simulink library "Tire_Models"  (R2020b)
settings: Solver=VariableStepAuto  StartTime=0.0  StopTime=10.0  RelTol=1e-3
undefined symbols (not defined in the file): Vehicle, X, Y, Z
libraries: Tire_Delft x4, Tire_CFL x2, Tire_MFEval x2, Tire_MFSwift x2, Tire_Testrig_Post x2, $bdroot x2, sm_lib x2
Description:
  | Copyright 2020 The MathWorks, Inc.
settings Model: Creator=smiller  LastModifiedBy=smiller
settings DataIOCC: ReturnWorkspaceOutputs=off
settings DebuggingCC: ArithmeticOperatorsInVariantConditions=warning
settings SFSimCC: CustomCodeUndefinedFunction=UseInterfaceOnly

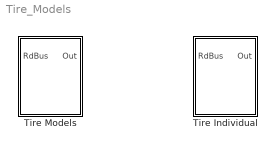
== system Tire_Models ==
  Tire Individual : Subsystem  Tag=PublishSubsystem  Variant=on  VariantControlMode=label  VariantControl=Variant1  LabelModeActiveChoice=MFEval  mask(Tire){popup_leftRight=Right, tir_index=1, Tire=Vehicle.Chassis.TireF, VariantLabel=Vehicle.Chassis.TireF.class.Value, InitTriggerDropdown=1}
      mask prompts: popup_leftRight "Left/Right"; tir_index "Tire Index"; Tire "Tire Parameters"; VariantLabel "Variant Label"; InitTriggerDropdown "Initialization Trigger Dropdown"
      mask help: Configurable tire model.
      mask init:
      | curblk = gcb;
      | 
      | % Set variant for this block
      | set_param(curblk,'LabelModeActiveChoice',VariantLabel);
      | 
      | tir_variant = get_param(gcb,'ActiveVariant');
      | if (popup_leftRight == 1)
      |     if(strcmp(tir_variant,'MFEval'))
      |         set_param([gcb '/MFEval'],'tir_side','1 left');
      |         set_param([gcb '/MFEval'],'popup_leftRight','Left');
      |     elseif(strcmp(tir_variant,'CFL'))
      |         set_param([gcb '/CFL'],'popup_leftRight','Left');
      |     elseif(strcmp(tir_variant,'Testrig_Post'))
      |         set_param([gcb '/Testrig Post'],'popup_leftRight','Left');
      |     elseif(strcmp(tir_variant,'Delft'))
      |         set_param([gcb '/Delft'],'tire_side_mode','(1xxx) left');
      |         set_param([gcb '/Delft'],'popup_leftRight','Left');
      |     elseif(strcmp(tir_variant,'MFSwift'))
      |         set_param([gcb '/MFSwift'],'tire_side_mode','(x1xxx) left');
      |         set_param([gcb '/MFSwift'],'popup_leftRight','Left');    
      |     end
      | elseif (popup_leftRight == 2)
      |     if(strcmp(tir_variant,'MFEval'))
      |         set_param([gcb '/MFEval'],'tir_side','2 right');
      |         set_param([gcb '/MFEval'],'popup_leftRight','Right');
      |     elseif(strcmp(tir_variant,'CFL'))
      |         set_param([gcb '/CFL'],'popup_leftRight','Right');
      |     elseif(strcmp(tir_variant,'Testrig_Post'))
      |         set_param([gcb '/Testrig Post'],'popup_leftRight','Right');        
      |     elseif(strcmp(tir_variant,'Delft'))
      |         set_param([gcb '/Delft'],'tire_side_mode','(2xxx) right');
      |         set_param([gcb '/Delft'],'popup_leftRight','Right');
      |     elseif(strcmp(tir_variant,'MFSwift'))
      |         set_param([gcb '/MFSwift'],'tire_side_mode','(x2xxx) right');
      |         set_param([gcb '/MFSwift'],'popup_leftRight','Right');    
      |     end
      | end
      | 
      | % Trigger Mask Initialization for
      | % variant subsystems below this level
      | sm_car_lib_maskInitTrigger(curblk);
      settings: AttributesFormatString=%<ActiveVariant>
      mask TypeOptions popup_leftRight: Left | Right
      mask TypeOptions InitTriggerDropdown: 0 | 1
      mask Display:
      | switch lower(get_param(gcb,'LabelModeActiveChoice'))
      |     case 'mfeval', image('sm_car_vehicle_tire_mfeval_IMAGE.png');
      |     case 'delft', image('sm_car_vehicle_tire_delft_IMAGE.png');
      |     case 'mfswift', image('sm_car_vehicle_tire_delft_IMAGE.png');
      |     case 'cpi', image('sm_car_vehicle_tire_delftcpi_IMAGE.png');
      |     case 'cfl', image('sm_car_vehicle_tire_cfl_IMAGE.png');
      |     case 'testrig_post', image('sm_car_vehicle_tire_testrig_IMAGE.png');
      | end
  Tire Models : Subsystem  Tag=PublishSubsystem  Variant=on  VariantControlMode=label  VariantControl=Variant1  LabelModeActiveChoice=MFEval  mask(Tire){popup_leftRight=Right, tir_index=1, Tire=Vehicle.Chassis.TireR, VariantLabel=Vehicle.Chassis.TireR.class.Value, InitTriggerDropdown=1}
      mask prompts: popup_leftRight "Left/Right"; tir_index "Tire Index"; Tire "Tire Parameters"; VariantLabel "Variant Label"; InitTriggerDropdown "Initialization Trigger Dropdown"
      mask help: Configurable tire model.
      mask init:
      | curblk = gcb;
      | 
      | % Set variant for this block 
      | set_param(curblk,'LabelModeActiveChoice',VariantLabel);
      | 
      | tir_variant = get_param(gcb,'ActiveVariant');
      | if (popup_leftRight == 1)
      |     rhs_tire = 1;
      |     if(strcmp(tir_variant,'MFEval'))
      |         set_param([gcb '/MFEval'],'tir_side','1 left');
      |         set_param([gcb '/MFEval'],'popup_leftRight','Left');
      |     elseif(strcmp(tir_variant,'Tire2x'))
      |         set_param([gcb '/Tire2x'],'popup_leftRight','Left');
      |     elseif(strcmp(tir_variant,'CFL'))
      |         set_param([gcb '/CFL'],'popup_leftRight','Left');
      |     elseif(strcmp(tir_variant,'Testrig_Post'))
      |         set_param([gcb '/Testrig Post'],'popup_leftRight','Left');
      |     elseif(strcmp(tir_variant,'Delft'))
      |         set_param([gcb '/Delft'],'tire_side_mode','(1xxx) left');
      |         set_param([gcb '/Delft'],'popup_leftRight','Left');
      |     elseif(strcmp(tir_variant,'MFSwift'))
      |         set_param([gcb '/MFSwift'],'tire_side_mode','(x1xxx) left');
      |         set_param([gcb '/MFSwift'],'popup_leftRight','Left');
      |     end
      | elseif (popup_leftRight == 2)
      |     rhs_tire = -1;
      |     if(strcmp(tir_variant,'MFEval'))
      |         set_param([gcb '/MFEval'],'tir_side','2 right');
      |         set_param([gcb '/MFEval'],'popup_leftRight','Right');
      |     elseif(strcmp(tir_variant,'Tire2x'))
      |         set_param([gcb '/Tire2x'],'popup_leftRight','Right');
      |     elseif(strcmp(tir_variant,'CFL'))
      |         set_param([gcb '/CFL'],'popup_leftRight','Right');
      |     elseif(strcmp(tir_variant,'Testrig_Post'))
      |         set_param([gcb '/Testrig Post'],'popup_leftRight','Right');
      |     elseif(strcmp(tir_variant,'Delft'))
      |         set_param([gcb '/Delft'],'tire_side_mode','(2xxx) right');
      |         set_param([gcb '/Delft'],'popup_leftRight','Right');
      |     elseif(strcmp(tir_variant,'MFSwift'))
      |         set_param([gcb '/MFSwift'],'tire_side_mode','(x2xxx) right');
      |         set_param([gcb '/MFSwift'],'popup_leftRight','Right');
      |     end
      | end
      | 
      | % Trigger Mask Initialization for 
      | % variant subsystems below this level
      | sm_car_lib_maskInitTrigger(curblk);
      settings: AttributesFormatString=%<ActiveVariant>
      mask TypeOptions popup_leftRight: Left | Right
      mask TypeOptions InitTriggerDropdown: 0 | 1
      mask Display:
      | switch lower(get_param(gcb,'LabelModeActiveChoice'))
      |     case 'mfeval', image('sm_car_vehicle_tire_mfeval_IMAGE.png');
      |     case 'delft', image('sm_car_vehicle_tire_delft_IMAGE.png');
      |     case 'mfswift', image('sm_car_vehicle_tire_delft_IMAGE.png');
      |     case 'cpi', image('sm_car_vehicle_tire_delftcpi_IMAGE.png');
      |     case 'cfl', image('sm_car_vehicle_tire_cfl_IMAGE.png');
      |     case 'testrig_post', image('sm_car_vehicle_tire_testrig_IMAGE.png');
      |     case 'tire2x',
      |         switch lower(get_param([gcb '/Tire2x/Tire Inner'],'LabelModeActiveChoice'))
      |             case 'mfeval', image('sm_car_vehicle_tire_mfeval2x_IMAGE.png');
      |             case 'delft', image('sm_car_vehicle_tire_delft2x_IMAGE.png');
      |             case 'mfswift', image('sm_car_vehicle_tire_delft2x_IMAGE.png');
      |             case 'cfl', image('sm_car_vehicle_tire_cfl2x_IMAGE.png');
      |             case 'testrig', image('sm_car_vehicle_tire_testrig2x_IMAGE.png');
      |         end
      | end

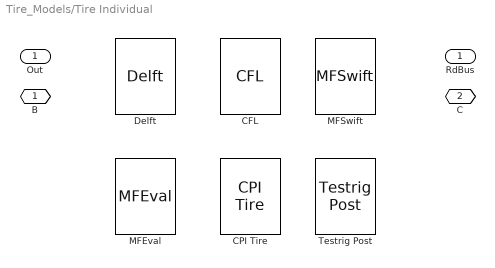
== system Tire_Models/Tire Individual ==
  RdBus : Inport
  CFL : Tire_CFL/CFL  VariantControl=CFL  popup_leftRight=Left  tire_radius=Tire.tire_radius.Value  rim_radius=Tire.rim_radius.Value  tire_width=Tire.tire_width.Value  rim_width=Tire.rim_width.Value  tyre_mass=Tire.tire_mass.Value  rim_mass=Tire.rim_mass.Value  tire_inertia=Tire.tire_J.Value  rim_inertia=Tire.rim_J.Value  plane_l=Tire.plane.l.Value  plane_w=Tire.plane.w.Value  k_contact=Tire.k.Value  b_contact=Tire.b.Value  mu_kinetic=Tire.mu_k.Value  mu_static=Tire.mu_s.Value  v_thr=Tire.v_thr.Value  TireBody=Tire.TireBody  InitTriggerDropdown=1  clr_tyre_cfl=Visual.Tire.clr  opc_tyre_cfl=Visual.Tire.opc  clr_rim_cfl=Visual.Rim.clr  opc_rim_cfl=Visual.Rim.opc
  CPI Tire : Tire_Delft/CPI Tire  VariantControl=CPI  idtyre=0
  Delft : Tire_Delft/Delft  VariantControl=Delft  idtyre=tir_index  rim_inertia=Tire.Inertia.Value  tir_name=Tire.tirFile.Value  rdf_name=Tire.roadFile.Value  tire_side_mode=(2xxx) right  tire_contact=Tire.Contact.Value  tire_dynamics=Tire.Dynamics.Value  tire_slip=Tire.Slip.Value  TireBody=Tire.TireBody  InitTriggerDropdown=1  popup_leftRight=Right  clr_tyre=Visual.Tire.clr  opc_tyre=Visual.Tire.opc  clr_rim=Visual.Rim.clr  opc_rim=Visual.Rim.opc
  MFEval : Tire_MFEval/MFEval  VariantControl=MFEval  tir_file=Tire.tirFile.Value  tir_side=2 right  tir_dynamics=Tire.Dynamics.Value  tir_mode=Tire.Mode.Value  TireBody=Tire.TireBody  InitTriggerDropdown=1  popup_leftRight=Right  clr_tyre=Visual.Tire.clr  opc_tyre=Visual.Tire.clr  clr_rim=Visual.Rim.clr  opc_rim=Visual.Rim.opc
  MFSwift : Tire_MFSwift/MFSwift  VariantControl=MFSwift  idtyre=tir_index  rim_inertia=Tire.Inertia.Value  tir_name=Tire.tirFile.Value  rdf_name=Tire.roadFile.Value  tire_side_mode=(x2xxx) right  tire_contact=Tire.Contact.Value  tire_dynamics=Tire.Dynamics.Value  tire_slip=Tire.Slip.Value  solver_enable=Tire.InternalSolver.Value  TireBody=Tire.TireBody  InitTriggerDropdown=1  popup_leftRight=Right  clr_tyre=Visual.Tire.clr  opc_tyre=Visual.Tire.opc  clr_rim=Visual.Rim.clr  opc_rim=Visual.Rim.opc
  Testrig Post : Tire_Testrig_Post/Testrig Post  VariantControl=Testrig_Post  popup_leftRight=Right  tire_k=Tire.K.Value  tire_b=Tire.b.Value  tire_radius=Tire.tire_radius.Value  rim_radius=Tire.rim_radius.Value  tire_width=Tire.tire_width.Value  rim_width=Tire.rim_width.Value  tyre_mass=Tire.tire_mass.Value  rim_mass=Tire.rim_mass.Value  tire_inertia=Tire.tire_J.Value  rim_inertia=Tire.rim_J.Value  TireBody=Tire.TireBody  platform=Scene.Testrig_Post  InitTriggerDropdown=1
  " B" : PMIOPort  Side=Right
  " C" : PMIOPort  Port=2  Side=Left
  " Out" : Outport  VectorParamsAs1DForOutWhenUnconnected=off

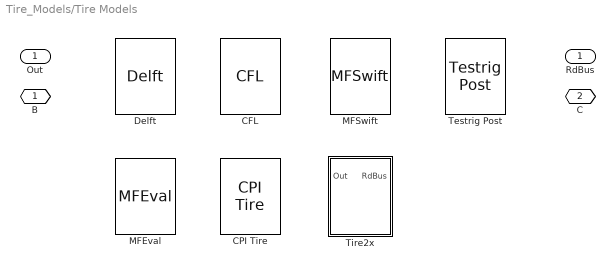
== system Tire_Models/Tire Models ==
  RdBus : Inport
  CFL : Tire_CFL/CFL  VariantControl=CFL  popup_leftRight=Right  tire_radius=Tire.tire_radius.Value  rim_radius=Tire.rim_radius.Value  tire_width=Tire.tire_width.Value  rim_width=Tire.rim_width.Value  tyre_mass=Tire.tire_mass.Value  rim_mass=Tire.rim_mass.Value  tire_inertia=Tire.tire_J.Value  rim_inertia=Tire.rim_J.Value  plane_l=Tire.plane.l.Value  plane_w=Tire.plane.w.Value  k_contact=Tire.k.Value  b_contact=Tire.b.Value  mu_kinetic=Tire.mu_k.Value  mu_static=Tire.mu_s.Value  v_thr=Tire.v_thr.Value  TireBody=Tire.TireBody  InitTriggerDropdown=1  clr_tyre_cfl=Visual.Tire.clr  opc_tyre_cfl=Visual.Tire.opc  clr_rim_cfl=Visual.Rim.clr  opc_rim_cfl=Visual.Rim.opc
  CPI Tire : Tire_Delft/CPI Tire  VariantControl=CPI  idtyre=0
  Delft : Tire_Delft/Delft  VariantControl=Delft  idtyre=tir_index  rim_inertia=Tire.Inertia.Value  tir_name=Tire.tirFile.Value  rdf_name=Tire.roadFile.Value  tire_side_mode=(2xxx) right  tire_contact=Tire.Contact.Value  tire_dynamics=Tire.Dynamics.Value  tire_slip=Tire.Slip.Value  TireBody=Tire.TireBody  InitTriggerDropdown=1  popup_leftRight=Right  clr_tyre=Visual.Tire.clr  opc_tyre=Visual.Tire.opc  clr_rim=Visual.Rim.clr  opc_rim=Visual.Rim.opc
  MFEval : Tire_MFEval/MFEval  VariantControl=MFEval  tir_file=Tire.tirFile.Value  tir_side=2 right  tir_dynamics=Tire.Dynamics.Value  tir_mode=Tire.Mode.Value  TireBody=Tire.TireBody  InitTriggerDropdown=1  popup_leftRight=Right  clr_tyre=Visual.Tire.clr  opc_tyre=Visual.Tire.opc  clr_rim=Visual.Rim.clr  opc_rim=Visual.Rim.opc
  MFSwift : Tire_MFSwift/MFSwift  VariantControl=MFSwift  idtyre=tir_index  rim_inertia=Tire.Inertia.Value  tir_name=Tire.tirFile.Value  rdf_name=Tire.roadFile.Value  tire_side_mode=(x2xxx) right  tire_contact=Tire.Contact.Value  tire_dynamics=Tire.Dynamics.Value  tire_slip=Tire.Slip.Value  solver_enable=Tire.InternalSolver.Value  TireBody=Tire.TireBody  InitTriggerDropdown=1  popup_leftRight=Right  clr_tyre=Visual.Tire.clr  opc_tyre=Visual.Tire.opc  clr_rim=Visual.Rim.clr  opc_rim=Visual.Rim.opc
  Testrig Post : Tire_Testrig_Post/Testrig Post  VariantControl=Testrig_Post  popup_leftRight=Right  tire_k=Tire.K.Value  tire_b=Tire.b.Value  tire_radius=Tire.tire_radius.Value  rim_radius=Tire.rim_radius.Value  tire_width=Tire.tire_width.Value  rim_width=Tire.rim_width.Value  tyre_mass=Tire.tire_mass.Value  rim_mass=Tire.rim_mass.Value  tire_inertia=Tire.tire_J.Value  rim_inertia=Tire.rim_J.Value  TireBody=Tire.TireBody  platform=Scene.Testrig_Post  InitTriggerDropdown=1
  Tire2x : Subsystem  VariantControl=Tire2x  mask{popup_leftRight=Right, tir_index=tir_index, TireInner=Tire.TireInner, TireOuter=Tire.TireOuter, InitTriggerDropdown=1}
      mask prompts: popup_leftRight "Left/Right"; tir_index "Tire Index"; TireInner "Tire Inner (structure)"; TireOuter "Tire Outer (structure)"; InitTriggerDropdown "Initialization Trigger Dropdown"
      mask init:
      | curblk = gcb;
      | 
      | if(popup_leftRight == 1)
      |     set_param([curblk '/Tire Inner'],'popup_leftRight','Left');
      |     set_param([curblk '/Tire Outer'],'popup_leftRight','Left');
      | elseif(popup_leftRight == 2)
      |     set_param([curblk '/Tire Inner'],'popup_leftRight','Right');
      |     set_param([curblk '/Tire Outer'],'popup_leftRight','Right');
      | end
      | 
      | % Trigger Mask Initialization for 
      | % variant subsystems below this level
      | sm_car_lib_maskInitTrigger(curblk);
      mask TypeOptions popup_leftRight: Left | Right
      mask TypeOptions InitTriggerDropdown: 0 | 1
      mask DialogControl cont_tire_mfeval Prompt: Tire
  " B" : PMIOPort  Side=Right
  " C" : PMIOPort  Port=2  Side=Left
  " Out" : Outport  VectorParamsAs1DForOutWhenUnconnected=off

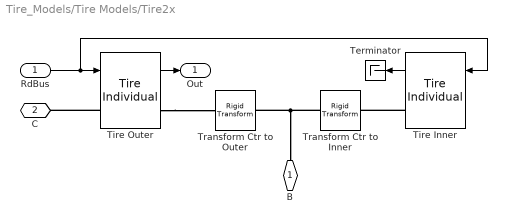
== system Tire_Models/Tire Models/Tire2x ==
  RdBus : Inport
  Terminator : Terminator
  Tire Inner : $bdroot/Tire Individual  Tag=PublishSubsystem  VariantControl=Variant1  LabelModeActiveChoice=MFEval  popup_leftRight=Right  tir_index=tir_index+10  Tire=TireInner  VariantLabel=TireInner.class.Value  InitTriggerDropdown=1
      settings: AttributesFormatString=%<ActiveVariant>
  Tire Outer : $bdroot/Tire Individual  Tag=PublishSubsystem  VariantControl=Variant1  LabelModeActiveChoice=MFEval  popup_leftRight=Right  tir_index=tir_index  Tire=TireOuter  VariantLabel=TireOuter.class.Value  InitTriggerDropdown=1
      settings: AttributesFormatString=%<ActiveVariant>
  Transform Ctr to Inner : sm_lib/Frames and Transforms/Rigid Transform  TranslationMethod=StandardAxis  TranslationStandardOffset=Tire.xOffset.Value/2*rhs_tire  TranslationLengthUnit=m  TranslationStandardAxis=-Z  TranslationCartesianOffset=[0 0 0]  TranslationROffset=0  TranslationROffsetUnits=m  TranslationZOffset=0  TranslationZOffsetUnits=m  TranslationThetaOffset=0  TranslationThetaOffsetUnits=deg  RotationMethod=None  RotationAngleUnits=deg  RotationStandardAxis=+Z  RotationAngle=0.0  RotationArbitraryAxis=[0 0 1]  FollAlignAxisA=+X  BaseAlignAxisA=+Y  FollAlignAxisB=+Y  BaseAlignAxisB=+Z  RotationSequenceAxes=FollowerAxes  RotationSequence=XYX  RotationSequenceAngles=[0 0 0]  RotationSequenceAnglesUnits=deg  RotationMatrix=[1 0 0; 0 1 0; 0 0 1]
  Transform Ctr to Outer : sm_lib/Frames and Transforms/Rigid Transform  TranslationMethod=StandardAxis  TranslationStandardOffset=Tire.xOffset.Value/2*rhs_tire  TranslationLengthUnit=m  TranslationStandardAxis=+Z  TranslationCartesianOffset=[0 0 0]  TranslationROffset=0  TranslationROffsetUnits=m  TranslationZOffset=0  TranslationZOffsetUnits=m  TranslationThetaOffset=0  TranslationThetaOffsetUnits=deg  RotationMethod=None  RotationAngleUnits=deg  RotationStandardAxis=+Z  RotationAngle=0.0  RotationArbitraryAxis=[0 0 1]  FollAlignAxisA=+X  BaseAlignAxisA=+Y  FollAlignAxisB=+Y  BaseAlignAxisB=+Z  RotationSequenceAxes=FollowerAxes  RotationSequence=XYX  RotationSequenceAngles=[0 0 0]  RotationSequenceAnglesUnits=deg  RotationMatrix=[1 0 0; 0 1 0; 0 0 1]
  B : PMIOPort  Side=Right
  C : PMIOPort  Port=2  Side=Left
  Out : Outport  VectorParamsAs1DForOutWhenUnconnected=off
  wires:
  RdBus/1 -> Tire Outer/1, Tire Inner/1
  Tire Outer/1 -> Out/1
  Tire Inner/1 -> Terminator/1
  connections:
  Transform Ctr to Inner/LConn1 -- B/RConn1 -- Transform Ctr to Outer/LConn1
  Tire Outer/LConn1 -- C/RConn1
  Tire Inner/RConn1 -- Transform Ctr to Inner/RConn1
  Tire Outer/RConn1 -- Transform Ctr to Outer/RConn1
